simulink model "lcl_pi"  (R2015a)
settings: Solver=ode45  StartTime=0.0  StopTime=.04  MaxStep=Ts/1000  RelTol=1e-3
values from neighbouring files (symbols this model uses):
  k1 = (beta^2 - a*(1 - k2) + k2)*Lfc/b    [Sim_lcl_pi.m]
  k2 = -2*beta + a + 1    [Sim_lcl_pi.m]
  ki = -Ka(5)    [Sim_lcl_fs.m]    (also in Sim_lcl_pi.m = k1 - k2*a*Lfc/b)
  kt = ki/(1 - beta)    [Sim_lcl_fs.m]    (also in Sim_lcl_pi.m = (1 - beta)*Lfc/b)
  sigmaNoise = 0*.1    (= 0)    [Sim_lcl_fs.m]    (also in Sim_lcl_pi.m)
  TNoise = Ts    (= 0.0002)    [Sim_lcl_fs.m]    (also in Sim_lcl_pi.m = 0.00015)
  Ts = 200e-6    (= 0.0002)    [Sim_lcl_fs.m]    (also in Sim_lcl_pi.m = 0.00015)
  Tsw = Ts    (= 0.0002)    [Sim_lcl_fs.m]    (also in Sim_lcl_pi.m = 0.00015)
  Udc = 350    [Sim_lcl_fs.m]    (also in Sim_lcl_pi.m)
  ug0 = ug0Act    (= 300)    [Sim_lcl_fs.m]    (also in Sim_lcl_pi.m)
  ug0Act = 300    [Sim_lcl_fs.m]    (also in Sim_lcl_pi.m)
  ui0 = ug0 + K*[0; ug0; 0; ug0]    [Sim_lcl_fs.m]    (also in Sim_lcl_pi.m = ug0 + k2*ug0)
  uMax = Udc    (= 350)    [Sim_lcl_fs.m]    (also in Sim_lcl_pi.m)
undefined symbols (not defined in the file): CfAct, LfcAct, LfgAct
libraries: simulink x2
settings Model: Creator=mhink  LastModifiedBy=mhinkkan
settings DataIOCC: SaveFormat=Dataset
settings HardwareCC: ProdBitPerPointer=64  ProdLargestAtomicFloat=Float  ProdIntDivRoundTo=Zero  ProdEndianess=LittleEndian  ProdHWDeviceType=Specified
settings GRTTargetCC: GeneratePreprocessorConditionals=Use local settings

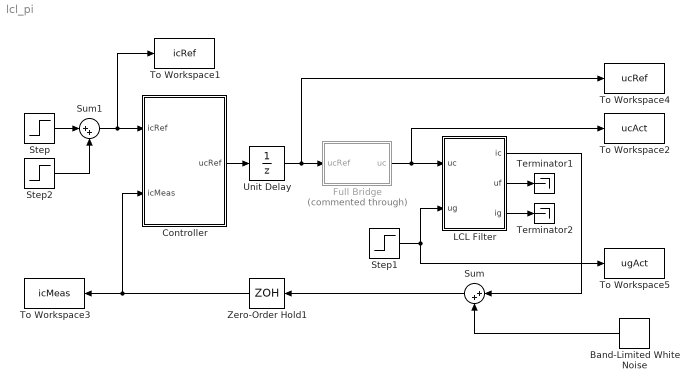
== system lcl_pi ==
  Band-Limited White Noise : simulink/Sources/Band-Limited White Noise  Cov=[sigmaNoise^2*TNoise]  Ts=TNoise  seed=[23341]
  Controller : Subsystem
  Full Bridge : Subsystem  Commented=through
  LCL Filter : Subsystem  mask{Lfc=LfcAct, Cf=CfAct, Lfg=LfgAct, ug0=ug0Act}
      mask prompts: Lfc "Converter-side inductance Lfc (H)"; Cf "Capacitance Cf (F)"; Lfg "Grid-side inductance Lfg (H)"; ug0 "Initial value ug0 (V)"
  Step : Step  Time=.002  After=10  SampleTime=Ts
  Step1 : Step  Time=.01  Before=ug0Act  After=200  SampleTime=0
  Step2 : Step  Time=.02  After=10  SampleTime=Ts
  Sum : Sum  Inputs=|++
  Sum1 : Sum  Inputs=|++
  Terminator1 : Terminator
  Terminator2 : Terminator
  To Workspace1 : ToWorkspace  VariableName=icRef  SaveFormat=Timeseries  SampleTime=-1
  To Workspace2 : ToWorkspace  VariableName=ucAct  SaveFormat=Timeseries  SampleTime=-1
  To Workspace3 : ToWorkspace  VariableName=icMeas  SaveFormat=Timeseries  SampleTime=-1
  To Workspace4 : ToWorkspace  VariableName=ucRef  SaveFormat=Timeseries  SampleTime=-1
  To Workspace5 : ToWorkspace  VariableName=ugAct  SaveFormat=Timeseries  SampleTime=Ts
  Unit Delay : UnitDelay  InitialCondition=ug0  SampleTime=Ts
  Zero-Order Hold1 : ZeroOrderHold  SampleTime=Ts
  wires:
  Controller/1(ucRef) -> Unit Delay/1
  Full Bridge/1(uc) -> LCL Filter/1(uc), To Workspace2/1
  Zero-Order Hold1/1 -> To Workspace3/1, Controller/2(icMeas)
  Step1/1 -> To Workspace5/1, LCL Filter/2(ug)
  Unit Delay/1 -> To Workspace4/1, Full Bridge/1(ucRef)
  LCL Filter/1(ic) -> Sum/1
  Sum/1 -> Zero-Order Hold1/1
  Band-Limited White Noise/1 -> Sum/2
  Step/1 -> Sum1/1
  Sum1/1 -> To Workspace1/1, Controller/1(icRef)
  Step2/1 -> Sum1/2
  LCL Filter/2(uf) -> Terminator1/1
  LCL Filter/3(ig) -> Terminator2/1

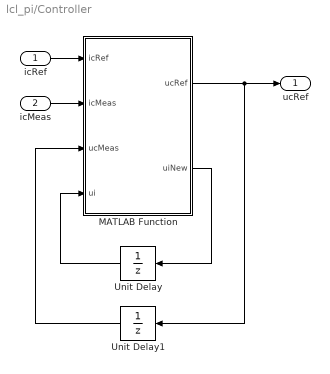
== system lcl_pi/Controller ==
  icRef : Inport
  icMeas : Inport  Port=2
  MATLAB Function : MATLAB Function  TreatAsAtomicUnit=on
      settings: PermitHierarchicalResolution=ParametersOnly
  Unit Delay : UnitDelay  InitialCondition=ui0  SampleTime=Ts
  Unit Delay1 : UnitDelay  InitialCondition=ug0  SampleTime=Ts
  ucRef : Outport
  wires:
  MATLAB Function/2(uiNew) -> Unit Delay/1
  icRef/1 -> MATLAB Function/1(icRef)
  MATLAB Function/1(ucRef) -> Unit Delay1/1, ucRef/1
  Unit Delay/1 -> MATLAB Function/4(ui)
  Unit Delay1/1 -> MATLAB Function/3(ucMeas)
  icMeas/1 -> MATLAB Function/2(icMeas)

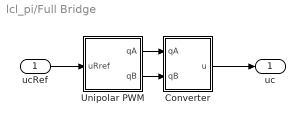
== system lcl_pi/Full Bridge ==
  ucRef : Inport
  Converter : Subsystem
  Unipolar PWM : Subsystem
  uc : Outport
  wires:
  Converter/1(u) -> uc/1
  Unipolar PWM/2(qB) -> Converter/2(qB)
  Unipolar PWM/1(qA) -> Converter/1(qA)
  ucRef/1 -> Unipolar PWM/1(uRref)

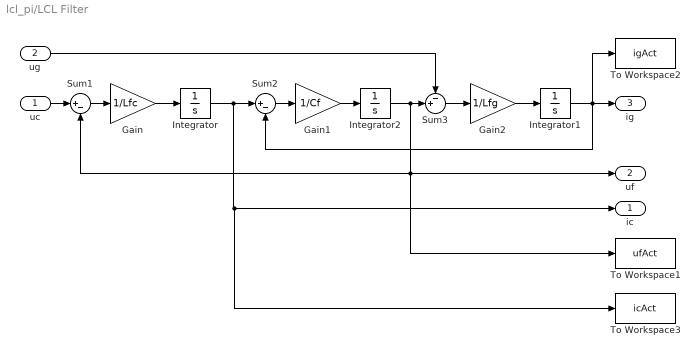
== system lcl_pi/LCL Filter ==
  uc : Inport
  ug : Inport  Port=2
  Gain : Gain  Gain=1/Lfc
  Gain1 : Gain  Gain=1/Cf
  Gain2 : Gain  Gain=1/Lfg
  Integrator : Integrator
  Integrator1 : Integrator
  Integrator2 : Integrator  InitialCondition=ug0
  Sum1 : Sum  Inputs=|+-
  Sum2 : Sum  Inputs=|+-
  Sum3 : Sum  Inputs=-+|
  To Workspace1 : ToWorkspace  VariableName=ufAct  SaveFormat=Timeseries  SampleTime=-1
  To Workspace2 : ToWorkspace  VariableName=igAct  SaveFormat=Timeseries  SampleTime=-1
  To Workspace3 : ToWorkspace  VariableName=icAct  SaveFormat=Timeseries  SampleTime=-1
  ic : Outport
  uf : Outport  Port=2
  ig : Outport  Port=3
  wires:
  uc/1 -> Sum1/1
  Sum1/1 -> Gain/1
  Gain/1 -> Integrator/1
  Integrator/1 -> To Workspace3/1, ic/1, Sum2/1
  Sum2/1 -> Gain1/1
  Gain1/1 -> Integrator2/1
  Sum3/1 -> Gain2/1
  Integrator1/1 -> To Workspace2/1, Sum2/2, ig/1
  Gain2/1 -> Integrator1/1
  Integrator2/1 -> To Workspace1/1, Sum1/2, uf/1, Sum3/2
  ug/1 -> Sum3/1

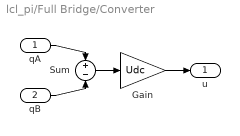
== system lcl_pi/Full Bridge/Converter ==
  qA : Inport
  qB : Inport  Port=2
  Gain : Gain  Gain=Udc
  Sum : Sum  Inputs=+|-
  u : Outport
  wires:
  qA/1 -> Sum/1
  qB/1 -> Sum/2
  Gain/1 -> u/1
  Sum/1 -> Gain/1

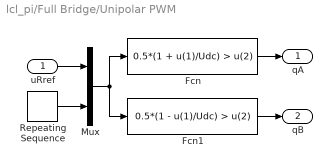
== system lcl_pi/Full Bridge/Unipolar PWM ==
  uRref : Inport
  Fcn : Fcn  Expr=0.5*(1 + u(1)/Udc) > u(2)
  Fcn1 : Fcn  Expr=0.5*(1 - u(1)/Udc) > u(2)
  Mux : Mux  Inputs=2
  Repeating Sequence : simulink/Sources/Repeating Sequence  rep_seq_t=Tsw*[0 0.5 1]  rep_seq_y=[1 0 1]
  qA : Outport
  qB : Outport  Port=2
  wires:
  uRref/1 -> Mux/1
  Mux/1 -> Fcn1/1, Fcn/1
  Repeating Sequence/1 -> Mux/2
  Fcn/1 -> qA/1
  Fcn1/1 -> qB/1

== matlab function lcl_pi/Controller/MATLAB Function ==
  data: icRef input size=1; ucRef output size=1; icMeas input; ucMeas input; ui input size=1; uiNew output size=1; uMax parameter; kt parameter; k1 parameter; ki parameter; k2 parameter
function [ucRef,uiNew] = fcn(icRef,icMeas, ucMeas,ui,uMax,kt,k1, ki, k2)

ucRefIdeal = kt*icRef - k1*icMeas - k2*ucMeas + ui;

% Limit the output
ucRef = ucRefIdeal;
if(ucRef > uMax)
    ucRef = uMax;
elseif(ucRef < -uMax)
    ucRef = -uMax;
end

% Update the integrator state. Last term is the antiwindup.
uiNew = ui + ki*((icRef - icMeas) + (ucRef - ucRefIdeal)/kt);
